simulink model "L6"  (R2015a)
settings: Solver=ode45  StartTime=0.0  StopTime=10.0  RelTol=1e-3
settings Model: Creator=User  LastModifiedBy=User

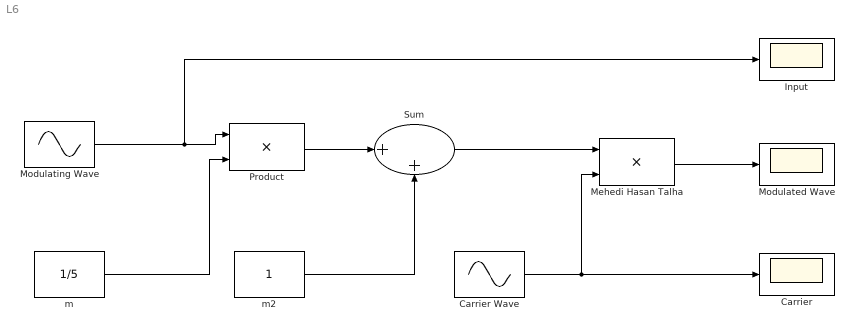
== system L6 ==
  Carrier : Scope
      settings: SaveName=ScopeData2
  Carrier Wave : Sin  Amplitude=5  Frequency=2*pi*25  SampleTime=1/5000
  Input : Scope
  Mehedi Hasan Talha : Product
  "Modulated Wave " : Scope
  Modulating Wave : Sin  Frequency=2*pi  SampleTime=1/5000
  Product : Product
  Sum : Sum  Inputs=|++
  m : Constant  Value=1/5
  m2 : Constant
  wires:
  Modulating Wave/1 -> Input/1, Product/1
  m/1 -> Product/2
  Product/1 -> Sum/1
  m2/1 -> Sum/2
  Sum/1 -> Mehedi Hasan Talha/1
  Carrier Wave/1 -> Carrier/1, Mehedi Hasan Talha/2
  Mehedi Hasan Talha/1 -> "Modulated Wave "/1
